simulink model "LAB5T3"  (R2018b)
settings: Solver=VariableStepAuto  StartTime=0.0  StopTime=400  RelTol=1e-3
settings Model: Creator=aloisia  LastModifiedBy=aloisia

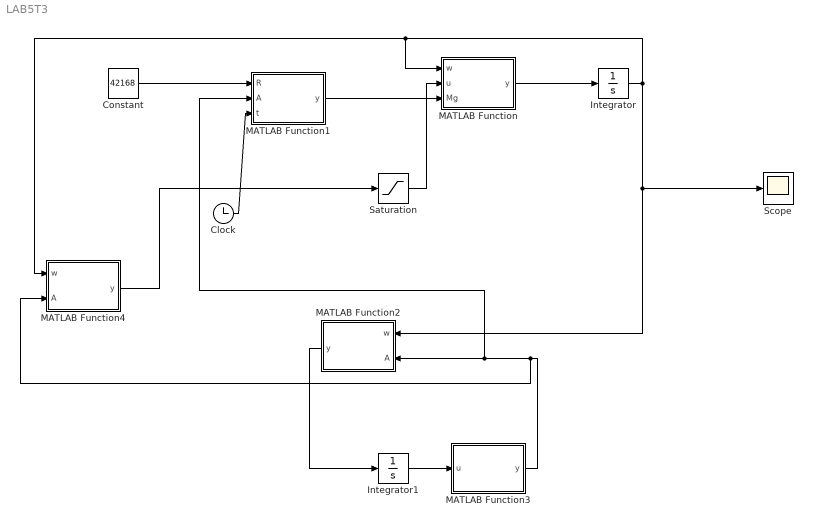
== system LAB5T3 ==
  Clock : Clock
  Constant : Constant  Value=42168
  Integrator : Integrator  InitialCondition=[0.1; 0.1; 0.1]
  Integrator1 : Integrator  InitialCondition=[-0.782 0 -0.6233;-0.6233 0 -0.782;0 -1 0]
  MATLAB Function : MATLAB Function  TreatAsAtomicUnit=on
  MATLAB Function1 : MATLAB Function  TreatAsAtomicUnit=on
  MATLAB Function2 : MATLAB Function  TreatAsAtomicUnit=on
  MATLAB Function3 : MATLAB Function  TreatAsAtomicUnit=on
  MATLAB Function4 : MATLAB Function  TreatAsAtomicUnit=on
  Saturation : Saturate  UpperLimit=5e-3  LowerLimit=-5e-3
  Scope : Scope
  wires:
  MATLAB Function/1(y) -> Integrator/1
  MATLAB Function1/1(y) -> MATLAB Function/3(Mg)
  Clock/1 -> MATLAB Function1/3(t)
  Integrator1/1 -> MATLAB Function3/1(u)
  MATLAB Function3/1(y) -> MATLAB Function4/2(A), MATLAB Function1/2(A), MATLAB Function2/2(A)
  MATLAB Function2/1(y) -> Integrator1/1
  Constant/1 -> MATLAB Function1/1(R)
  Integrator/1 -> MATLAB Function2/1(w), Scope/1, MATLAB Function4/1(w), MATLAB Function/1(w)
  MATLAB Function4/1(y) -> Saturation/1
  Saturation/1 -> MATLAB Function/2(u)

== matlab function LAB5T3/MATLAB Function1 ==
  data: R input; A input; y output; t input
function y = GravityGrad(R,A,t)

%Data
mu = 398600;
n2 = mu/ R^3;
n = sqrt(n2);
J1=0.01;
J2=0.05;
J3=0.07;

Aln = [cos(n*t) sin(n*t) 0; -sin(n*t) cos(n*t) 0;0 0 1];
Abl = A* Aln';
c = Abl *[1;0;0];

Mg = zeros (3,1);
Mg(1) = 3*n2*(J3-J2)/J1*c(3)*c(2);
Mg(2) = 3*n2*(J1-J3)/J2*c(1)*c(3);
Mg(3) = 3*n2*(J2-J1)/J3*c(2)*c(1);

y = Mg;
end

== matlab function LAB5T3/MATLAB Function ==
  data: w input; u input; y output; Mg input
function y = Euler(w,u,Mg)
%First laboratory

%Datas
J1=0.01;
J2=0.05;
J3=0.07;

omx=w(1);
omy=w(2);
omz=w(3);

%Formula
omxdot=(J2-J3)/J1*omy*omz + u(1)/J1 + Mg(1)/J1;
omydot=(J3-J1)/J2*omx*omz + u(2)/J2 + Mg(2)/J2;
omzdot=(J1-J2)/J3*omy*omx + u(3)/J3 + Mg(3)/J3;

y=[omxdot; omydot; omzdot];

end

== matlab function LAB5T3/MATLAB Function2 ==
  data: w input; y output; A input
function y = Kinematic(w,A)

W=[0 -w(3) w(2);w(2) 0 -w(1);-w(2) w(1) 0];
Adot=-W*A;
y=Adot;
end

== matlab function LAB5T3/MATLAB Function3 ==
  data: u input; y output
function y = Orthonorm(u)

t=abs(trace(eye(3)-u'*u));

 while t>0.000000001 
    A=(1.5)*u-u*u'*0.5*u;
    t=abs(trace(eye(3)-A'*A));
    u=A;
   
 end

y=u;
end

== matlab function LAB5T3/MATLAB Function4 ==
  data: w input; A input; y output
function y = control_law(w,A)

J1=0.01;
J2=0.05;
J3=0.07;

J = diag([J1,J2,J3]);

% Set k1 and k2 due to have a faster stabilization
k1 = 0.01;
k2 = 0.01;

K = k1 * J;
C = k2 * J;

% Set control matrix Ac
Ac = eye(3);
% Set error matrix Ae
Ae = A*(Ac');
d = (Ae'- Ae);
e = [d(3,2);d(1,3);d(2,1)];

u = - K*e - C*w;

y=u;
